simulink model "vehicule_fuzzy_controller"  (R2024a)
settings: Solver=VariableStepAuto  StartTime=0.0  StopTime=25.0  RelTol=1e-3
libraries: simulink x3, fuzblock x2
settings Model: Creator=idial068  LastModifiedBy=odaal085

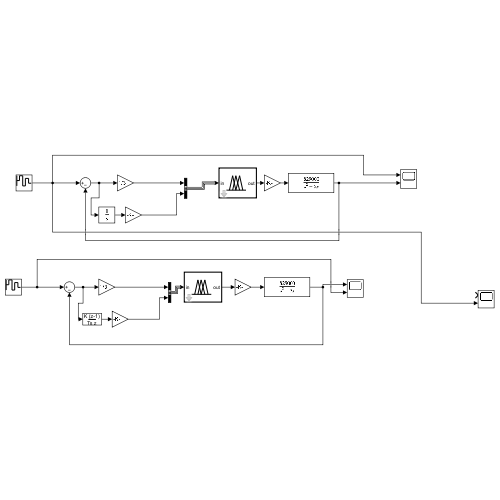
[thumbnail: Simulink's stored preview of the top-level diagram]
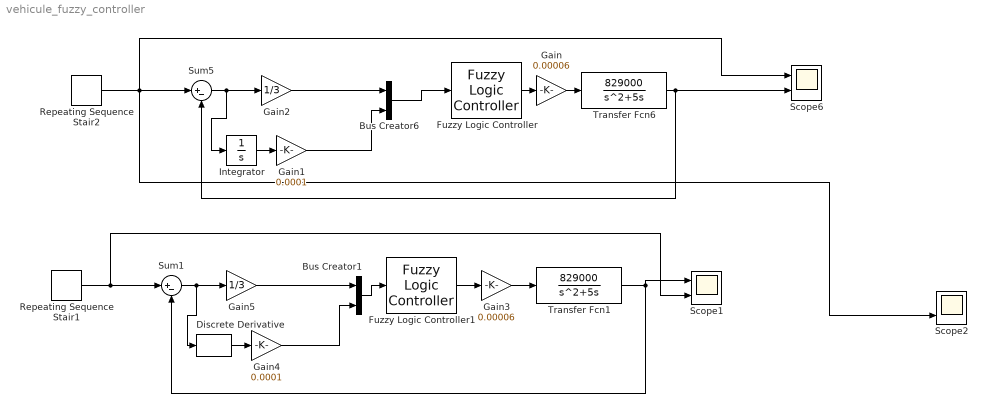
== system vehicule_fuzzy_controller ==
  Bus Creator1 : BusCreator  Inputs=2
  Bus Creator6 : BusCreator  Inputs=2
  Discrete Derivative : simulink/Discrete/Discrete Derivative  gainval=1.0  ICPrevScaledInput=0.0  OutMin=[]  OutMax=[]  OutDataType=fixdt(1, 16)  OutScaling=2^-10  DoSatur=off
  Fuzzy Logic Controller : fuzblock/Fuzzy Logic  Controller  FIS='FLC.fis'  OutputSampleNumber=101  DataType=double  FuzzifiedInputs=off  RuleFiringStrengths=off  RuleOutputs=off  AggregatedOutputs=off  SimulateUsing=Interpreted execution  OutOfRangeInputValueMessage=warning  NoRuleFiredMessage=warning  EmptyOutputFuzzySetMessage=warning
  Fuzzy Logic Controller1 : fuzblock/Fuzzy Logic  Controller  FIS='FLC.fis'  OutputSampleNumber=101  DataType=double  FuzzifiedInputs=off  RuleFiringStrengths=off  RuleOutputs=off  AggregatedOutputs=off  SimulateUsing=Interpreted execution  OutOfRangeInputValueMessage=warning  NoRuleFiredMessage=warning  EmptyOutputFuzzySetMessage=warning
  Gain : Gain  Gain=0.00006
  Gain1 : Gain  Gain=0.0001
  Gain2 : Gain  Gain=1/3
  Gain3 : Gain  Gain=0.00006
  Gain4 : Gain  Gain=0.0001
  Gain5 : Gain  Gain=1/3
  Integrator : Integrator
  Repeating Sequence Stair1 : simulink/Sources/Repeating Sequence Stair  OutValues=[20 30 10 25 15].'  tsamp=5  OutMin=[]  OutMax=[]  OutDataTypeStr=double  OutputDataTypeScalingMode=double  OutDataType=fixdt(0,8)  ConRadixGroup=Best Precision: Vector-wise  OutScaling=2^-12
  Repeating Sequence Stair2 : simulink/Sources/Repeating Sequence Stair  OutValues=[20 30 10 25 15].'  tsamp=5  OutMin=[]  OutMax=[]  OutDataTypeStr=double  OutputDataTypeScalingMode=double  OutDataType=fixdt(0,8)  ConRadixGroup=Best Precision: Vector-wise  OutScaling=2^-12
  Scope1 : Scope  NumInputPorts=2
  Scope2 : Scope  NumInputPorts=2
  Scope6 : Scope  NumInputPorts=2
  Sum1 : Sum  Inputs=|+-
  Sum5 : Sum  Inputs=|+-
  Transfer Fcn1 : TransferFcn  Numerator=[829000]  Denominator=[1 5 0]
  Transfer Fcn6 : TransferFcn  Numerator=[829000]  Denominator=[1 5 0]
  wires:
  Integrator/1 -> Gain1/1
  Transfer Fcn6/1 -> Scope6/2, Sum5/2
  Fuzzy Logic Controller/1 -> Gain/1
  Gain/1 -> Transfer Fcn6/1
  Gain3/1 -> Transfer Fcn1/1
  Discrete Derivative/1 -> Gain4/1
  Fuzzy Logic Controller1/1 -> Gain3/1
  Transfer Fcn1/1 -> Scope1/1, Sum1/2
  Repeating Sequence Stair1/1 -> Scope1/2, Sum1/1
  Repeating Sequence Stair2/1 -> Scope6/1, Scope2/2, Sum5/1
  Sum1/1 -> Discrete Derivative/1, Gain5/1
  Sum5/1 -> Integrator/1, Gain2/1
  Gain1/1 -> Bus Creator6/2
  Gain5/1 -> Bus Creator1/1
  Gain4/1 -> Bus Creator1/2
  Bus Creator1/1 -> Fuzzy Logic Controller1/1
  Bus Creator6/1 -> Fuzzy Logic Controller/1
  Gain2/1 -> Bus Creator6/1
